simulink model "kalman"  (R2017b)
settings: Solver=FixedStepAuto  StartTime=0.0  StopTime=10  FixedStep=0.001  RelTol=1e-3
values from neighbouring files (symbols this model uses):
  A = [Z I Z ... (first row only)    [LIMPMatrices.m]
  B = [B_u B_d]    [LIMPMatrices.m]
  C = [I Z -I/omega^2 ... (first row only)    [LIMPMatrices.m]
  D = [D_u D_d]    [LIMPMatrices.m]
undefined symbols (not defined in the file or in its folder): A_kal, Bu_kal, Cm_kal, L_kal, M_kal
libraries: mpclib x1, simulink x1
settings Model: Creator=francesco  LastModifiedBy=francesco
settings RTWCC: GenCodeOnly=on  GenerateReport=on  Toolchain=GNU gcc/g++ v4.4.x | gmake (64-bit Linux)  BuildConfiguration=Faster Runs  LaunchReport=on  TargetLang=C++
settings GRTTargetCC: TargetLangStandard=C++03 (ISO)  MatFileLogging=off  MultiInstanceERTCode=on  CodeInterfacePackaging=C++ class

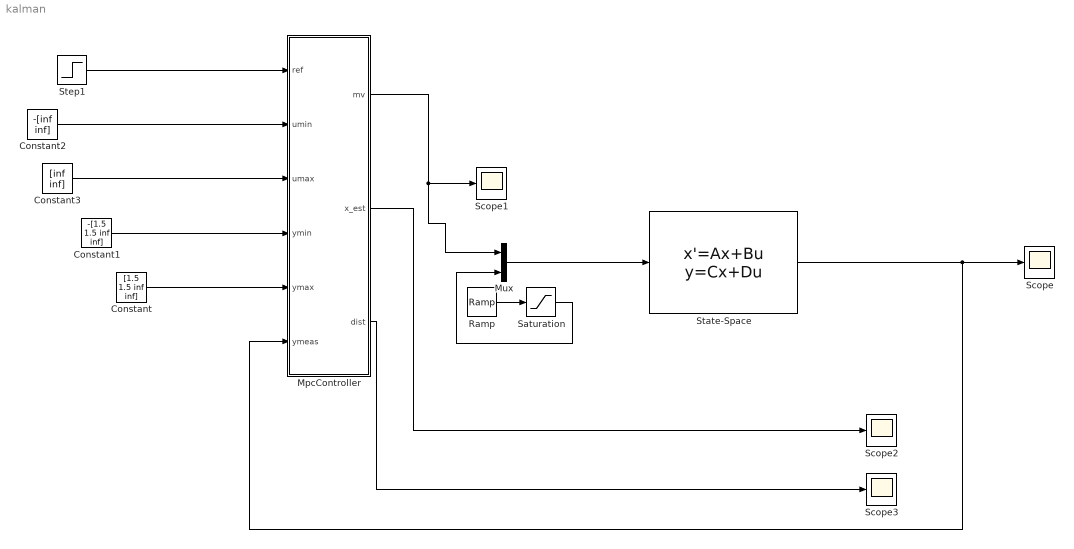
== system kalman ==
  Constant : Constant  Value=[1.5 1.5 inf inf]
  Constant1 : Constant  Value=-[1.5 1.5 inf inf]
  Constant2 : Constant  Value=-[inf inf]
  Constant3 : Constant  Value=[inf inf]
  MpcController : Subsystem  TreatAsAtomicUnit=on  SystemSampleTime=0.001
  Mux : Mux  Inputs=2
  Ramp : simulink/Sources/Ramp  slope=[1 0]  start=2  X0=0
  Saturation : Saturate  UpperLimit=1
  Scope{,1..3} (4 alike) : Scope
  State-Space : StateSpace  A=A  B=B  C=C  D=D  InitialCondition=0
  Step1 : Step  Time=0  Before=[0 0 0 0]  After=[0 0 0 0]  SampleTime=0.001
  wires:
  Mux/1 -> State-Space/1
  Ramp/1 -> Saturation/1
  Saturation/1 -> Mux/2
  State-Space/1 -> MpcController/6(ymeas), Scope/1
  MpcController/1(mv) -> Mux/1, Scope1/1
  Step1/1 -> MpcController/1(ref)
  Constant2/1 -> MpcController/2(umin)
  Constant3/1 -> MpcController/3(umax)
  Constant1/1 -> MpcController/4(ymin)
  Constant/1 -> MpcController/5(ymax)
  MpcController/2(x_est) -> Scope2/1
  MpcController/3(dist) -> Scope3/1

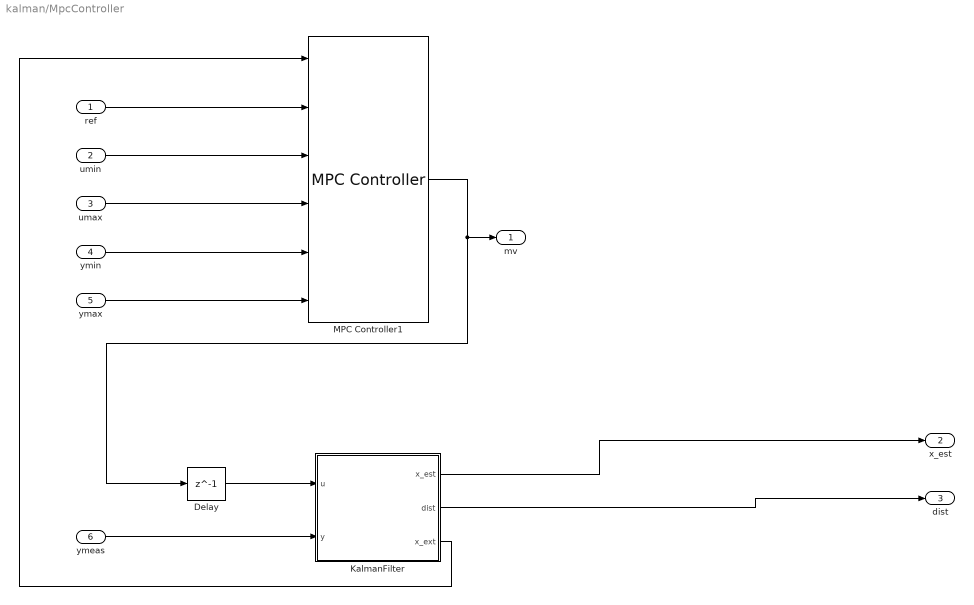
== system kalman/MpcController ==
  ref : Inport
  umin : Inport  Port=2
  umax : Inport  Port=3
  ymin : Inport  Port=4
  ymax : Inport  Port=5
  ymeas : Inport  Port=6
  Delay : Delay  DelayLength=1
  KalmanFilter : Subsystem  TreatAsAtomicUnit=on
  MPC Controller1 : mpclib/MPC Controller  SCDEnableBlockLinearizationSpecification=on  mpcobj=mpc1  is_multiple=0  enable_value=0  return_u0=off  ref_from_ws=off  ref_signal_name=[]  ref_preview=off  md_from_ws=off  md_signal_name=[]  md_preview=off  from_project=off  project_file=MPCtask.mat  md_inport=off  mv_inport=off  cost_outport=off  return_sequence=off  return_qpstatus=off  return_state=off  state_inport=on  lims_inport=on  cc_inport=off  ywt_inport=off  is_designfromscratch=0  uwt_inport=off  duwt_inport=off  rhoeps_inport=off  uref_inport=off  n_ts=0.05  n_p=30  n_mv=2  n_md=0  n_ud=2  n_mo=4  n_uo=0  BlockDataType=double  SampleTimeInherited=on  switch_inport=off
  mv : Outport
  x_est : Outport  Port=2
  dist : Outport  Port=3
  wires:
  ymax/1 -> MPC Controller1/6
  umax/1 -> MPC Controller1/4
  KalmanFilter/3(x_ext) -> MPC Controller1/1
  umin/1 -> MPC Controller1/3
  ymin/1 -> MPC Controller1/5
  KalmanFilter/2(dist) -> dist/1
  ymeas/1 -> KalmanFilter/2(y)
  ref/1 -> MPC Controller1/2
  KalmanFilter/1(x_est) -> x_est/1
  MPC Controller1/1 -> mv/1, Delay/1
  Delay/1 -> KalmanFilter/1(u)

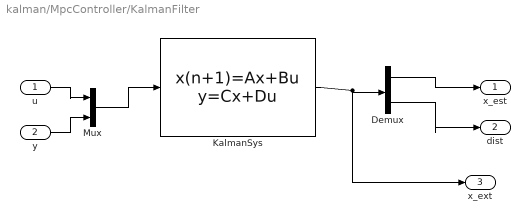
== system kalman/MpcController/KalmanFilter ==
  u : Inport
  y : Inport  Port=2
  Demux : Demux  Outputs=[8 2]
  KalmanSys : DiscreteStateSpace  A=A_kal-L_kal*Cm_kal  B=[Bu_kal L_kal]  C=eye(10) - M_kal*Cm_kal  D=[zeros(10,2) M_kal]  SampleTime=0.001
  Mux : Mux  Inputs=2
  x_est : Outport
  dist : Outport  Port=2
  x_ext : Outport  Port=3
  wires:
  u/1 -> Mux/1
  y/1 -> Mux/2
  Mux/1 -> KalmanSys/1
  Demux/1 -> x_est/1
  Demux/2 -> dist/1
  KalmanSys/1 -> x_ext/1, Demux/1
